simulink model "demo_simulink"  (R2016a)
settings: Solver=FixedStepAuto  StartTime=0.0  StopTime=50.0  FixedStep=0.01  RelTol=1e-3
settings Model: Creator=aula  LastModifiedBy=aula

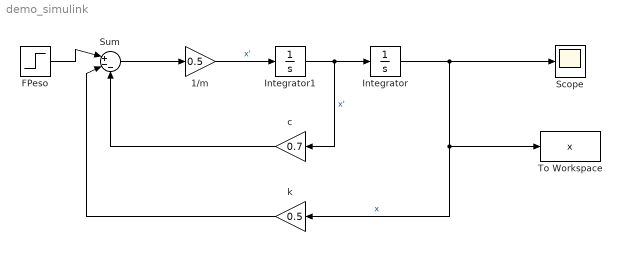
== system demo_simulink ==
  "1/m " : Gain  Gain=0.5
  "FPeso " : Step  SampleTime=0
  Integrator : Integrator
  Integrator1 : Integrator
  Scope : Scope
  Sum : Sum  Inputs=|+--
  To Workspace : ToWorkspace  VariableName=x  SampleTime=-1
  c : Gain  Gain=0.7
  k : Gain  Gain=0.5
  wires:
  c/1 -> Sum/3
  Sum/1 -> "1/m "/1
  "1/m "/1 -> Integrator1/1  "x'"
  Integrator1/1 -> c/1, Integrator/1  "x'"
  Integrator/1 -> To Workspace/1, k/1, Scope/1  "x"
  k/1 -> Sum/2
  "FPeso "/1 -> Sum/1
